simulink model "two_2"  (R2014a)
settings: Solver=ode45  StartTime=0.0  StopTime=30  RelTol=1e-3
settings Model: Creator=Павел  LastModifiedBy=Павел

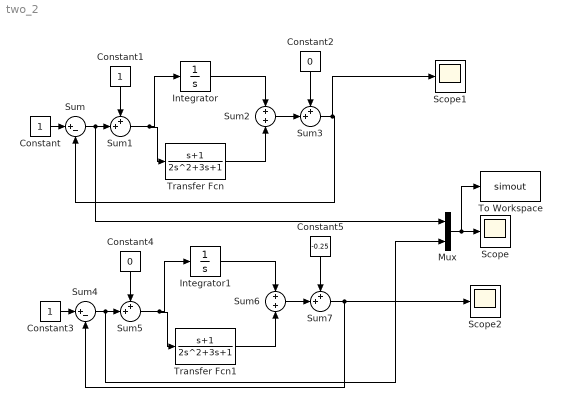
== system two_2 ==
  Constant : Constant
  Constant1 : Constant
  Constant2 : Constant  Value=0
  Constant3 : Constant
  Constant4 : Constant  Value=0
  Constant5 : Constant  Value=-0.25
  Integrator : Integrator  InitialCondition=1
  Integrator1 : Integrator  InitialCondition=1
  Mux : Mux  Inputs=2
  Scope : Scope
  Scope1 : Scope
  Scope2 : Scope
      settings: SaveName=ScopeData2
  Sum : Sum  Inputs=|+-
  Sum{1,3,5,7} (4 alike) : Sum  Inputs=++|
  Sum2 : Sum  Inputs=+|+
  Sum4 : Sum  Inputs=|+-
  Sum6 : Sum  Inputs=+|+
  To Workspace : ToWorkspace  VariableName=simout  SaveFormat=Timeseries  SampleTime=-1
  Transfer Fcn : TransferFcn  Numerator=[1 1]  Denominator=[2 3 1]
  Transfer Fcn1 : TransferFcn  Numerator=[1 1]  Denominator=[2 3 1]
  wires:
  Constant/1 -> Sum/1
  Sum/1 -> Mux/1, Sum1/2
  Constant1/1 -> Sum1/1
  Sum1/1 -> Transfer Fcn/1, Integrator/1
  Integrator/1 -> Sum2/1
  Transfer Fcn/1 -> Sum2/2
  Sum2/1 -> Sum3/2
  Constant2/1 -> Sum3/1
  Sum3/1 -> Scope1/1, Sum/2
  Constant3/1 -> Sum4/1
  Sum4/1 -> Mux/2, Sum5/2
  Constant4/1 -> Sum5/1
  Sum5/1 -> Integrator1/1, Transfer Fcn1/1
  Integrator1/1 -> Sum6/1
  Transfer Fcn1/1 -> Sum6/2
  Sum6/1 -> Sum7/2
  Constant5/1 -> Sum7/1
  Sum7/1 -> Sum4/2, Scope2/1
  Mux/1 -> To Workspace/1, Scope/1
